simulink model "HindmarshRose"  (R2014b)
settings: Solver=ode45  StartTime=0.0  StopTime=10.0  RelTol=1e-3
values from neighbouring files (symbols this model uses):
  a = 0.95    [Run_Aizawa.m]    (also in Run_Arneodo.m = -5.5; Run_Chen.m = 33; Run_Chua.m = 15.6; Run_Chua_4D.m = 0.03)
  b = 0.7    [Run_Aizawa.m]    (also in Run_Arneodo.m = 3.5; Run_Chen.m = 3; Run_Chua.m = 28; Run_Duffing.m = 100)
  c = -1    [Run_Arneodo.m]    (also in Run_Chen.m = 25; Run_Chua_4D.m = -1.2; Run_Dadras.m = 2; Run_HindmarshRose.m = 1)
  d = 4 * 1e-3    (= 0.004)    [Run_Belousov_Zhabotinsky.m]    (also in Run_HindmarshRose.m = 5; Run_Qi_4D.m = 0.6; Run_Roessler_4D.m = 0.05)
  I = 3    [Run_HindmarshRose.m]
  r = 1.7    [Run_Dadras.m]    (also in Run_HindmarshRose.m = 0.01; Run_Lorenz.m = 100; Script_Lorenz.m = 28)
  s = 3.5    [Run_Aizawa.m]    (also in Run_Chua_4D.m = 0.75; Run_Duffing.m = 0.2; Run_HindmarshRose.m = 4; Run_Lorenz.m = 10)
  xR = -8/5    (= -1.6)    [Run_HindmarshRose.m]
undefined symbols (not defined in the file or in its folder): param
settings Model: Creator=Arek  LastModifiedBy=Arek

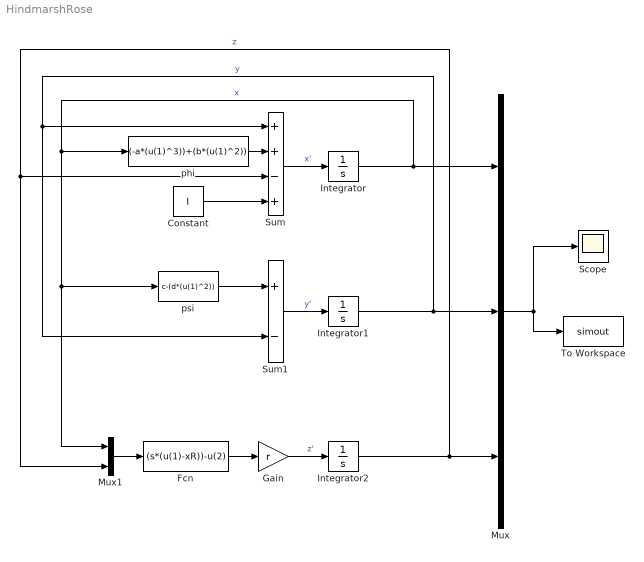
== system HindmarshRose ==
  Constant : Constant  Value=I
  Fcn : Fcn  Expr=(s*(u(1)-xR))-u(2)
  Gain : Gain  Gain=r
  Integrator : Integrator  InitialCondition=param.ic(1)
  Integrator1 : Integrator  InitialCondition=param.ic(2)
  Integrator2 : Integrator  InitialCondition=param.ic(3)
  Mux : Mux  Inputs=3
  Mux1 : Mux  Inputs=2
  Scope : Scope
      settings: ShowLegends=on  TimeRange=0.05  YMin=-6  YMax=2
  Sum : Sum  Inputs=++-+
  Sum1 : Sum  Inputs=+-
  To Workspace : ToWorkspace  VariableName=simout  SaveFormat=Timeseries  SampleTime=-1
  phi : Fcn  Expr=(-a*(u(1)^3))+(b*(u(1)^2))
  psi : Fcn  Expr=c-(d*(u(1)^2))
  wires:
  Gain/1 -> Integrator2/1  "z'"
  Sum1/1 -> Integrator1/1  "y'"
  Sum/1 -> Integrator/1  "x'"
  Integrator/1 -> Mux1/1, psi/1, phi/1, Mux/1  "x"
  Integrator1/1 -> Sum/1, Sum1/2, Mux/2  "y"
  Integrator2/1 -> Mux1/2, Sum/3, Mux/3  "z"
  Mux/1 -> Scope/1, To Workspace/1
  phi/1 -> Sum/2
  Constant/1 -> Sum/4
  psi/1 -> Sum1/1
  Fcn/1 -> Gain/1
  Mux1/1 -> Fcn/1
